simulink model "test_fmu_arch"  (R2022a)
settings: Solver=FixedStepAuto  StartTime=0.0  StopTime=10.0  RelTol=1e-3
settings Model: Creator=lordx  LastModifiedBy=lordx
settings OptimizationCC: UseDivisionForNetSlopeComputation=on  OptimizeBlockIOStorage=off  InitFltsAndDblsToZero=on  EfficientMapNaN2IntZero=off  BufferReusableBoundary=off
settings HardwareCC: TargetBitPerPointer=64  TargetBitPerSizeT=64  TargetBitPerPtrDiffT=64  TargetLongLongMode=on  TargetIntDivRoundTo=Zero  TargetEndianess=LittleEndian  TargetWordSize=64  TargetHWDeviceType=MATLAB Host  ProdEqTarget=off
settings RTWCC: Description=FMU based on GRT (Functional Mock-up Unit)  SystemTargetFile=grtfmi.tlc  GenerateMakefile=off  TemplateMakefile=none  GenerateReport=on  RetainRTWFile=on
settings CodeAppCC: ForceParamTrailComments=on  StateflowObjectComments=on  MATLABSourceComments=on
settings STFCustomTargetCC: TargetLangStandard=C99 (ISO)  CombineOutputUpdateFcns=on  GRTInterface=off  SystemTargetFile=grtfmi.tlc
settings GRTTargetCC: ParMdlRefBuildCompliant=off  CompOptLevelCompliant=off  ConcurrentExecutionCompliant=off  MatFileLogging=off  CPPClassGenCompliant=off  UseToolchainInfoCompliant=off  RTWCAPISignals=on  RTWCAPIParams=on  RTWCAPIStates=on  RTWCAPIRootIO=on

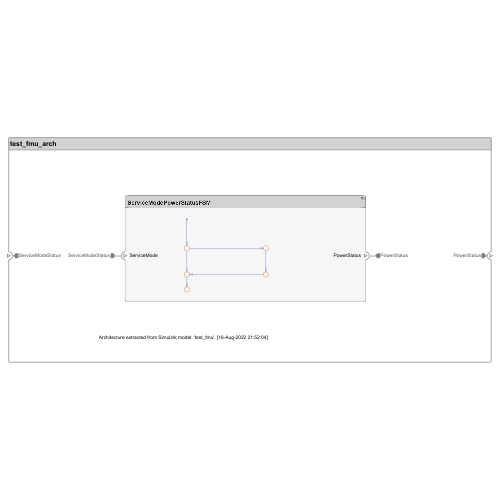
[thumbnail: Simulink's stored preview of the top-level diagram]
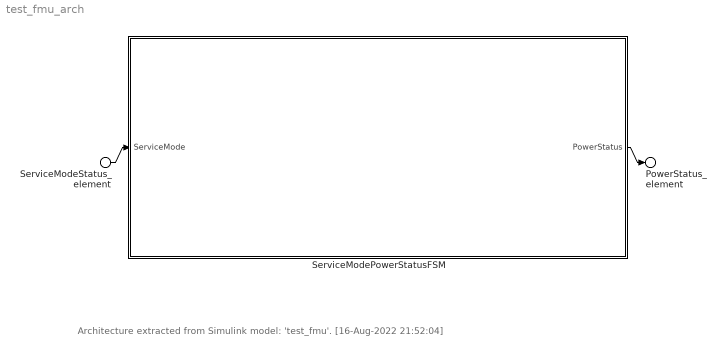
== system test_fmu_arch ==
  note: Architecture extracted from Simulink model: 'test_fmu'. [16-Aug-2022 21:52:04]
  ServiceModeStatus_element : Inport  PortName=ServiceModeStatus
  ServiceModePowerStatusFSM : Stateflow chart  TreatAsAtomicUnit=on
      settings: PortSchema="{\"entries\":[{\"content\":{\"headerSize\":26,\"margin\":15,\"minimumSpacing\":25,\"sides\":[{\"content\":{\"connectorIds\":[\"In1\"]},\"type\":\"ConnectorPlacement.EquallySpacedRectSide\",\"uuid\":\"ee8f242f-9245-4014-bba5-adee5f5da91a\"},{\"content\":{\"connectorIds\":[\"Out1\"],\"side\":\"RIGHT\"},\"type\":\"ConnectorPlacement.EquallySpacedRectSide\",\"uuid\":\"e7114069-b988-4f0c-ba11-6473b42aed19\"},{\"content\":{\"connectorIds\":[],\"side\":\"TOP\"},\"type\":\"ConnectorPlacement.EquallySpacedRectSide\",\"uuid\":\"de8c4458-881d-4ed2-bfd6-5abfa066daf4\"}]},\"type\":\"ConnectorPlacement.EquallySpacedConnector\",\"uuid\":\"4aa5a02c-2aa6-4ec9-a99b-15b940474f40\"}],\"packageUris\":[\"http://schema.mathworks.com/mf0/Connector/R2020b\"],\"version\":\"1.0\"}"
  PowerStatus_element : Outport  PortName=PowerStatus
  wires:
  ServiceModeStatus_element/1 -> ServiceModePowerStatusFSM/1(ServiceMode)
  ServiceModePowerStatusFSM/1(PowerStatus) -> PowerStatus_element/1

== stateflow chart test_fmu_arch/ServiceModePowerStatusFSM ==
  (default) -> (junction 8) : /* Service Mode State Machine */
  (junction 8) -> (junction 4) [order 1] : [ServiceMode != 0]
  (junction 8) -> (junction 1) [order 2] : {PowerStatus = 0;}
  (junction 4) -> (junction 9) : {PowerStatus = 1;}
  (junction 9) -> (junction 1) : [ServiceMode == 0]
  (junction 1) -> (junction 6)
  data: ServiceMode input; PowerStatus output double
